simulink model "HeatX2DShapeOpts"  (R2015a)
settings: Solver=FixedStepDiscrete  StartTime=0.0  StopTime=tsim  FixedStep=dt  RelTol=1e-3
values from neighbouring files (symbols this model uses):
  Cp2d = Cp*ones(length(y0),length(x))    [run_HeatX2DShapeOpts.m]
  hb = 0.05    [run_HeatX2DShapeOpts.m]
  hl = 0.05    [run_HeatX2DShapeOpts.m]
  hr = 0.05    [run_HeatX2DShapeOpts.m]
  ht = 0.05    [run_HeatX2DShapeOpts.m]
  k2d = k*ones(length(y0),length(x))    [run_HeatX2DShapeOpts.m]
  m = length(y0)    [run_HeatX2DShapeOpts.m]
  n = length(x)    [run_HeatX2DShapeOpts.m]
  rho2d = rho*ones(length(y0),length(x))    [run_HeatX2DShapeOpts.m]
  Tb = 850    [run_HeatX2DShapeOpts.m]
  Tl = 850    [run_HeatX2DShapeOpts.m]
  Tr = 850    [run_HeatX2DShapeOpts.m]
  Tt = 850    [run_HeatX2DShapeOpts.m]
libraries: lib_Conduction_2DCondADI x3
settings Model: Creator=jlkratz  LastModifiedBy=jlkratz

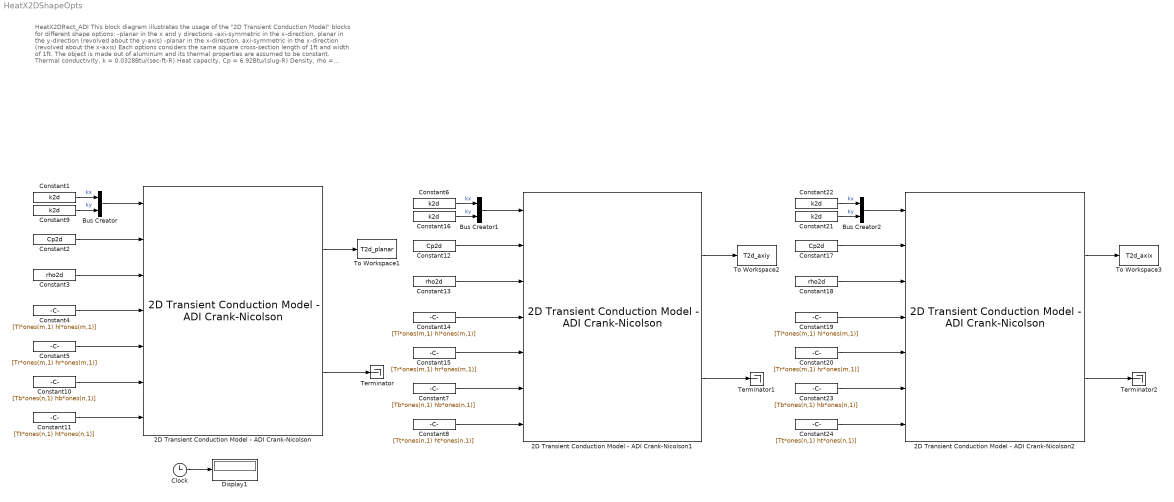
== system HeatX2DShapeOpts ==
  note: HeatX2DRect_ADI
      |
      | This block diagram illustrates the usage of the "2D Transient Conduction Model" blocks for different shape options:
      | -planar in the x and y directions
      | -axi-symmetric in the x-direction, planar in the y-direction (revolved about the y-axis)
      | -planar in the x-direction, axi-symmetric in the x-direction (revolved about the x-axis)
      |
      | Each options considers the same square cross-section length of 1ft and width of 1ft. The object is made
      | out of aluminum and its thermal properties are assumed to be constant.
      | Thermal conductivity, k = 0.0328Btu/(sec-ft-R)
      | Heat capacity, Cp = 6.92Btu/(slug-R)
      | Density, rho = 5.24slug/ft^3
      | The plate is at an initial temperature of 550R throughout. It is heated on all sides by convection via a fluid with a
      | temperature of 850R and a heat transfer coefficient of 0.05Btu/(sec-ft^2-R)
  2D Transient Conduction Model - ADI Crank-Nicolson : lib_Conduction_2DCondADI/2D Transient Conduction Model - ADI Crank-Nicolson  T0_M=T02d  dt_M=dt  x_M=x  y_M=y0  shape_M=Planar in both directions  convL_M=on  radL_M=off  condL_M=off  convR_M=on  radR_M=off  condR_M=off  convB_M=on  radB_M=off  condB_M=off  convT_M=on  radT_M=off  condT_M=off  BN_M=double(gcb)
  2D Transient Conduction Model - ADI Crank-Nicolson1 : lib_Conduction_2DCondADI/2D Transient Conduction Model - ADI Crank-Nicolson  T0_M=T02d  dt_M=dt  x_M=x  y_M=y0  shape_M=Axi-Symmetric in x-direction, Planar in y-direction  convL_M=on  radL_M=off  condL_M=off  convR_M=on  radR_M=off  condR_M=off  convB_M=on  radB_M=off  condB_M=off  convT_M=on  radT_M=off  condT_M=off  BN_M=double(gcb)
  2D Transient Conduction Model - ADI Crank-Nicolson2 : lib_Conduction_2DCondADI/2D Transient Conduction Model - ADI Crank-Nicolson  T0_M=T02d  dt_M=dt  x_M=x  y_M=y0  shape_M=Planar in x-direction, Axi-symmetric in y-direction  convL_M=on  radL_M=off  condL_M=off  convR_M=on  radR_M=off  condR_M=off  convB_M=on  radB_M=off  condB_M=off  convT_M=on  radT_M=off  condT_M=off  BN_M=double(gcb)
  Bus Creator : BusCreator  Inputs=2
  Bus Creator1 : BusCreator  Inputs=2
  Bus Creator2 : BusCreator  Inputs=2
  Clock : Clock
  Constant{1,6,9,16,21..22} (6 alike) : Constant  Value=k2d
  Constant10 : Constant  Value=[Tb*ones(n,1) hb*ones(n,1)]
  Constant11 : Constant  Value=[Tt*ones(n,1) ht*ones(n,1)]
  Constant12 : Constant  Value=Cp2d
  Constant13 : Constant  Value=rho2d
  Constant14 : Constant  Value=[Tl*ones(m,1) hl*ones(m,1)]
  Constant15 : Constant  Value=[Tr*ones(m,1) hr*ones(m,1)]
  Constant17 : Constant  Value=Cp2d
  Constant18 : Constant  Value=rho2d
  Constant19 : Constant  Value=[Tl*ones(m,1) hl*ones(m,1)]
  Constant2 : Constant  Value=Cp2d
  Constant20 : Constant  Value=[Tr*ones(m,1) hr*ones(m,1)]
  Constant23 : Constant  Value=[Tb*ones(n,1) hb*ones(n,1)]
  Constant24 : Constant  Value=[Tt*ones(n,1) ht*ones(n,1)]
  Constant3 : Constant  Value=rho2d
  Constant4 : Constant  Value=[Tl*ones(m,1) hl*ones(m,1)]
  Constant5 : Constant  Value=[Tr*ones(m,1) hr*ones(m,1)]
  Constant7 : Constant  Value=[Tb*ones(n,1) hb*ones(n,1)]
  Constant8 : Constant  Value=[Tt*ones(n,1) ht*ones(n,1)]
  Display1 : Display
  Terminator : Terminator
  Terminator1 : Terminator
  Terminator2 : Terminator
  To Workspace1 : ToWorkspace  VariableName=T2d_planar  SaveFormat=Timeseries  SampleTime=-1
  To Workspace2 : ToWorkspace  VariableName=T2d_axiy  SaveFormat=Timeseries  SampleTime=-1
  To Workspace3 : ToWorkspace  VariableName=T2d_axix  SaveFormat=Timeseries  SampleTime=-1
  wires:
  Constant1/1 -> Bus Creator/1  "kx"
  Constant9/1 -> Bus Creator/2  "ky"
  Bus Creator/1 -> 2D Transient Conduction Model - ADI Crank-Nicolson/1
  Constant2/1 -> 2D Transient Conduction Model - ADI Crank-Nicolson/2
  Constant3/1 -> 2D Transient Conduction Model - ADI Crank-Nicolson/3
  Constant11/1 -> 2D Transient Conduction Model - ADI Crank-Nicolson/7
  Constant10/1 -> 2D Transient Conduction Model - ADI Crank-Nicolson/6
  2D Transient Conduction Model - ADI Crank-Nicolson/1 -> To Workspace1/1
  2D Transient Conduction Model - ADI Crank-Nicolson/2 -> Terminator/1
  Constant4/1 -> 2D Transient Conduction Model - ADI Crank-Nicolson/4
  Constant5/1 -> 2D Transient Conduction Model - ADI Crank-Nicolson/5
  Clock/1 -> Display1/1
  Constant6/1 -> Bus Creator1/1  "kx"
  Constant16/1 -> Bus Creator1/2  "ky"
  Bus Creator1/1 -> 2D Transient Conduction Model - ADI Crank-Nicolson1/1
  Constant12/1 -> 2D Transient Conduction Model - ADI Crank-Nicolson1/2
  Constant13/1 -> 2D Transient Conduction Model - ADI Crank-Nicolson1/3
  Constant8/1 -> 2D Transient Conduction Model - ADI Crank-Nicolson1/7
  Constant7/1 -> 2D Transient Conduction Model - ADI Crank-Nicolson1/6
  2D Transient Conduction Model - ADI Crank-Nicolson1/1 -> To Workspace2/1
  2D Transient Conduction Model - ADI Crank-Nicolson1/2 -> Terminator1/1
  Constant14/1 -> 2D Transient Conduction Model - ADI Crank-Nicolson1/4
  Constant15/1 -> 2D Transient Conduction Model - ADI Crank-Nicolson1/5
  Constant22/1 -> Bus Creator2/1  "kx"
  Constant21/1 -> Bus Creator2/2  "ky"
  Bus Creator2/1 -> 2D Transient Conduction Model - ADI Crank-Nicolson2/1
  Constant17/1 -> 2D Transient Conduction Model - ADI Crank-Nicolson2/2
  Constant18/1 -> 2D Transient Conduction Model - ADI Crank-Nicolson2/3
  Constant24/1 -> 2D Transient Conduction Model - ADI Crank-Nicolson2/7
  Constant23/1 -> 2D Transient Conduction Model - ADI Crank-Nicolson2/6
  2D Transient Conduction Model - ADI Crank-Nicolson2/1 -> To Workspace3/1
  2D Transient Conduction Model - ADI Crank-Nicolson2/2 -> Terminator2/1
  Constant19/1 -> 2D Transient Conduction Model - ADI Crank-Nicolson2/4
  Constant20/1 -> 2D Transient Conduction Model - ADI Crank-Nicolson2/5
